simulink model "PSCelecv_2"  (R2020b)
settings: Solver=VariableStepAuto  StartTime=0.0  StopTime=100.0  RelTol=1e-3
undefined symbols (not defined in the file): sigbuilder_block
settings Model: Creator=colpari  LastModifiedBy=colpari

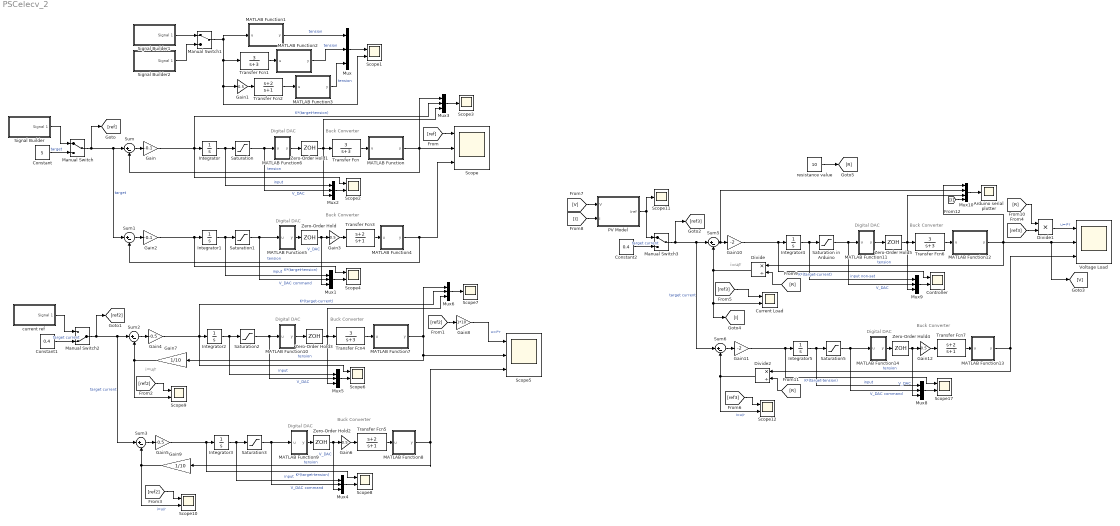
== system PSCelecv_2 ==
  note: i=u/r
  note: Digital DAC
  note: Digital DAC
  note: Buck Converter
  note: Buck Converter
  note: Buck Converter
  note: Digital DAC
  note: Buck Converter
  note: Digital DAC
  note: Buck Converter
  note: Digital DAC
  note: Digital DAC
  note: Buck Converter
  note: i=u/r
  Arduino serial plotter : Scope
  Constant : Constant  Value=5
  Constant1 : Constant  Value=0.4
  Constant2 : Constant  Value=0.4
  Controller : Scope  NumInputPorts=2
  Current Load : Scope  NumInputPorts=2
  Divide : Product  Inputs=*/
  Divide1 : Product  Inputs=**
  Divide2 : Product  Inputs=*/
  Gain : Gain  Gain=-0.1
  Gain{1,3,6,12} (4 alike) : Gain  Gain=0.5
  Gain10 : Gain  Gain=-2
  Gain11 : Gain  Gain=-2
  Gain2 : Gain  Gain=-0.1
  Gain4 : Gain  Gain=-0.5
  Gain5 : Gain  Gain=-0.5
  Gain7 : Gain  Gain=1/10
  Gain8 : Gain  Gain=1*10
  Gain9 : Gain  Gain=1/10
  Integrator{,1..5} (6 alike) : Integrator
  MATLAB Function : MATLAB Function  TreatAsAtomicUnit=on
  MATLAB Function1 : MATLAB Function  TreatAsAtomicUnit=on
  MATLAB Function10 : MATLAB Function  TreatAsAtomicUnit=on
  MATLAB Function11 : MATLAB Function  TreatAsAtomicUnit=on
  MATLAB Function12 : MATLAB Function  TreatAsAtomicUnit=on
  MATLAB Function13 : MATLAB Function  TreatAsAtomicUnit=on
  MATLAB Function14 : MATLAB Function  TreatAsAtomicUnit=on
  MATLAB Function2 : MATLAB Function  TreatAsAtomicUnit=on
  MATLAB Function3 : MATLAB Function  TreatAsAtomicUnit=on
  MATLAB Function4 : MATLAB Function  TreatAsAtomicUnit=on
  MATLAB Function5 : MATLAB Function  TreatAsAtomicUnit=on
  MATLAB Function6 : MATLAB Function  TreatAsAtomicUnit=on
  MATLAB Function7 : MATLAB Function  TreatAsAtomicUnit=on
  MATLAB Function8 : MATLAB Function  TreatAsAtomicUnit=on
  MATLAB Function9 : MATLAB Function  TreatAsAtomicUnit=on
  Manual Switch : ManualSwitch
  Manual Switch1 : ManualSwitch
  Manual Switch2 : ManualSwitch  CurrentSetting=0
  Manual Switch3 : ManualSwitch
  Mux{,1..6,8..9} (9 alike) : Mux  Inputs=3
  Mux10 : Mux
  PV Model : Subsystem
  Saturation{,1..3} (4 alike) : Saturate  UpperLimit=5  LowerLimit=1
  Saturation in Arduino : Saturate  UpperLimit=4.8  LowerLimit=0.2
  Saturation5 : Saturate  UpperLimit=4.8  LowerLimit=0.2
  Scope : Scope  NumInputPorts=3
  Scope{1..2,4,6,8..10,12,17} (9 alike) : Scope  NumInputPorts=2
  Scope11 : Scope
  Scope3 : Scope
  Scope5 : Scope  NumInputPorts=3
  Scope7 : Scope
  Signal Builder : Subsystem  Tag=STV Subsys  LoadFcn=sigbuilder_block('load');  StartFcn=sigbuilder_block('start');  StopFcn=sigbuilder_block('stop');  ClipboardFcn=sigbuilder_block('clipboard');  mask(Sigbuilder block){tuvar=[0:10]}
      mask help: Simulink:masks:SigbuilderBlock_MD
      mask init:
      | if ~strcmp(get_param(bdroot(gcbh),'SimulationStatus'),'stopped') tuvar = sigbuilder_block('maskInit'); end
      settings: CopyFcn=sigbuilder_block('copy');  DeleteFcn=sigbuilder_block('delete');  ModelCloseFcn=sigbuilder_block('modelClose');  PreSaveFcn=sigbuilder_block('preSave');  PauseFcn=sigbuilder_block('pause');  ContinueFcn=sigbuilder_block('continue');  NameChangeFcn=sigbuilder_block('namechange');  OpenFcn=sigbuilder_block('open',[337.5 87.75 550.5 399.75 ]);  CloseFcn=sigbuilder_block('close');
      mask Display: plot(0, 0, 100, 100,[2, 2, 32, 32, 2], [68, 8, 8, 68, 68],[32, 2], [38, 38], [32, 19, 2],[53, 60, 44], [32, 17, 17, 2],[16, 16, 31, 31]);txt = getActiveGroup(gcbh);text(2, 100, txt,'verticalAlignment', 'top');
  Signal Builder1 : Subsystem  Tag=STV Subsys  LoadFcn=sigbuilder_block('load');  StartFcn=sigbuilder_block('start');  StopFcn=sigbuilder_block('stop');  ClipboardFcn=sigbuilder_block('clipboard');  mask(Sigbuilder block){tuvar=[0:10]}
      mask help: Simulink:masks:SigbuilderBlock_MD
      mask init:
      | if ~strcmp(get_param(bdroot(gcbh),'SimulationStatus'),'stopped') tuvar = sigbuilder_block('maskInit'); end
      settings: CopyFcn=sigbuilder_block('copy');  DeleteFcn=sigbuilder_block('delete');  ModelCloseFcn=sigbuilder_block('modelClose');  PreSaveFcn=sigbuilder_block('preSave');  PauseFcn=sigbuilder_block('pause');  ContinueFcn=sigbuilder_block('continue');  NameChangeFcn=sigbuilder_block('namechange');  OpenFcn=sigbuilder_block('open',[437.6 199.2 550.4 400 ]);  CloseFcn=sigbuilder_block('close');
      mask Display: plot(0, 0, 100, 100,[2, 2, 32, 32, 2], [68, 8, 8, 68, 68],[32, 2], [38, 38], [32, 19, 2],[53, 60, 44], [32, 17, 17, 2],[16, 16, 31, 31]);txt = getActiveGroup(gcbh);text(2, 100, txt,'verticalAlignment', 'top');
  Signal Builder2 : Subsystem  Tag=STV Subsys  LoadFcn=sigbuilder_block('load');  StartFcn=sigbuilder_block('start');  StopFcn=sigbuilder_block('stop');  ClipboardFcn=sigbuilder_block('clipboard');  mask(Sigbuilder block){tuvar=[0:10]}
      mask help: Simulink:masks:SigbuilderBlock_MD
      mask init:
      | if ~strcmp(get_param(bdroot(gcbh),'SimulationStatus'),'stopped') tuvar = sigbuilder_block('maskInit'); end
      settings: CopyFcn=sigbuilder_block('copy');  DeleteFcn=sigbuilder_block('delete');  ModelCloseFcn=sigbuilder_block('modelClose');  PreSaveFcn=sigbuilder_block('preSave');  PauseFcn=sigbuilder_block('pause');  ContinueFcn=sigbuilder_block('continue');  NameChangeFcn=sigbuilder_block('namechange');  OpenFcn=sigbuilder_block('open',[337.5 87.75 550.5 399.75 ]);  CloseFcn=sigbuilder_block('close');
      mask Display: plot(0, 0, 100, 100,[2, 2, 32, 32, 2], [68, 8, 8, 68, 68],[32, 2], [38, 38], [32, 19, 2],[53, 60, 44], [32, 17, 17, 2],[16, 16, 31, 31]);txt = getActiveGroup(gcbh);text(2, 100, txt,'verticalAlignment', 'top');
  Sum{,1..3,5..6} (6 alike) : Sum  Inputs=|+-
  Transfer Fcn{,1,4,6} (4 alike) : TransferFcn  Numerator=[3]  Denominator=[1 3]
  Transfer Fcn{2..3,5,7} (4 alike) : TransferFcn  Numerator=[1 2]  Denominator=[1 1]
  Voltage Load : Scope  NumInputPorts=3
  Zero-Order Hold{,1..5} (6 alike) : ZeroOrderHold  SampleTime=0.05
  current ref : Subsystem  Tag=STV Subsys  LoadFcn=sigbuilder_block('load');  StartFcn=sigbuilder_block('start');  StopFcn=sigbuilder_block('stop');  ClipboardFcn=sigbuilder_block('clipboard');  mask(Sigbuilder block){tuvar=[0:10]}
      mask help: Simulink:masks:SigbuilderBlock_MD
      mask init:
      | if ~strcmp(get_param(bdroot(gcbh),'SimulationStatus'),'stopped') tuvar = sigbuilder_block('maskInit'); end
      settings: CopyFcn=sigbuilder_block('copy');  DeleteFcn=sigbuilder_block('delete');  ModelCloseFcn=sigbuilder_block('modelClose');  PreSaveFcn=sigbuilder_block('preSave');  PauseFcn=sigbuilder_block('pause');  ContinueFcn=sigbuilder_block('continue');  NameChangeFcn=sigbuilder_block('namechange');  OpenFcn=sigbuilder_block('open',[5.4 30 1141.2 594.6 ]);  CloseFcn=sigbuilder_block('close');
      mask Display: plot(0, 0, 100, 100,[2, 2, 32, 32, 2], [68, 8, 8, 68, 68],[32, 2], [38, 38], [32, 19, 2],[53, 60, 44], [32, 17, 17, 2],[16, 16, 31, 31]);txt = getActiveGroup(gcbh);text(2, 100, txt,'verticalAlignment', 'top');
  resistance value : Constant  Value=10
  wires:
  MATLAB Function/1(y) -> Mux3/1, Scope/2, Sum/2  "tension"
  Sum/1 -> Gain/1
  Transfer Fcn/1 -> MATLAB Function/1(u)
  Signal Builder/1(Signal 1) -> Manual Switch/1
  MATLAB Function1/1(y) -> Mux/1  "tension"
  Manual Switch1/1 -> Scope1/2, Gain1/1, Transfer Fcn1/1, MATLAB Function1/1(u)
  Transfer Fcn1/1 -> MATLAB Function2/1(u)
  MATLAB Function2/1(y) -> Mux/2  "tension"
  Constant/1 -> Manual Switch/2  "target"
  Gain/1 -> Mux3/2, Scope2/1, Integrator/1  "K*(target-tension)"
  Saturation/1 -> Mux2/2, MATLAB Function6/1(u)  "V_DAC"
  Mux/1 -> Scope1/1
  Integrator/1 -> Mux2/1, Saturation/1  "input"
  Signal Builder1/1(Signal 1) -> Manual Switch1/1
  Signal Builder2/1(Signal 1) -> Manual Switch1/2
  Transfer Fcn2/1 -> MATLAB Function3/1(u)
  MATLAB Function3/1(y) -> Mux/3  "tension"
  Gain1/1 -> Transfer Fcn2/1
  MATLAB Function4/1(y) -> Scope/3, Sum1/2  "tension"
  Saturation1/1 -> MATLAB Function5/1(u), Mux1/2  "V_DAC command"
  Sum1/1 -> Gain2/1
  Gain2/1 -> Scope4/1, Integrator1/1  "K*(target-tension)"
  Integrator1/1 -> Mux1/1, Saturation1/1  "input"
  Transfer Fcn3/1 -> MATLAB Function4/1(u)
  Manual Switch/1 -> [ref], Sum1/1, Sum/1  "target"
  Gain3/1 -> Transfer Fcn3/1
  [ref] -> Scope/1
  MATLAB Function5/1(y) -> Zero-Order Hold/1
  Zero-Order Hold/1 -> Mux1/3, Gain3/1  "V_DAC"
  MATLAB Function6/1(y) -> Zero-Order Hold1/1
  Zero-Order Hold1/1 -> Mux3/3, Mux2/3, Transfer Fcn/1
  Mux1/1 -> Scope4/2
  Mux2/1 -> Scope2/2
  Mux3/1 -> Scope3/1
  Transfer Fcn5/1 -> MATLAB Function8/1(u)
  Transfer Fcn4/1 -> MATLAB Function7/1(u)
  Mux5/1 -> Scope6/2
  Gain5/1 -> Scope8/1, Integrator3/1  "K*(target-tension)"
  MATLAB Function9/1(y) -> Zero-Order Hold2/1
  [ref2] -> Gain8/1
  Gain6/1 -> Transfer Fcn5/1
  Zero-Order Hold2/1 -> Mux4/3, Gain6/1  "V_DAC"
  Manual Switch2/1 -> [ref2], Sum3/1, Sum2/1  "target current"
  Gain4/1 -> Mux6/2, Scope6/1, Integrator2/1  "K*(target-current)"
  Saturation3/1 -> MATLAB Function9/1(u), Mux4/2  "V_DAC command"
  MATLAB Function8/1(y) -> Scope5/3, Gain9/1  "tension"
  Sum3/1 -> Gain5/1
  Constant1/1 -> Manual Switch2/2  "target current"
  Integrator2/1 -> Mux5/1, Saturation2/1  "input"
  Saturation2/1 -> Mux5/2, MATLAB Function10/1(u)  "V_DAC"
  Integrator3/1 -> Mux4/1, Saturation3/1  "input"
  MATLAB Function10/1(y) -> Zero-Order Hold3/1
  Mux4/1 -> Scope8/2
  current ref/1(Signal 1) -> Manual Switch2/1
  Sum2/1 -> Gain4/1
  MATLAB Function7/1(y) -> Gain7/1, Scope5/2, Mux6/1  "tension"
  Zero-Order Hold3/1 -> Mux6/3, Mux5/3, Transfer Fcn4/1
  Gain7/1 -> Scope9/2, Sum2/2
  Mux6/1 -> Scope7/1
  [ref2] -> Scope9/1
  Gain8/1 -> Scope5/1  "u=i*r"
  Gain9/1 -> Scope10/2, Sum3/2  "i=u/r"
  [ref2] -> Scope10/1
  [I] -> PV Model/2(I)
  [V] -> PV Model/1(V)
  [ref3] -> Current Load/1
  [ref3] -> Divide1/2
  Zero-Order Hold5/1 -> Mux10/3, Mux9/3, Transfer Fcn6/1
  PV Model/1(Iref) -> Manual Switch3/1, Scope11/1
  MATLAB Function11/1(y) -> Zero-Order Hold5/1
  MATLAB Function12/1(y) -> Divide/1, Mux10/1, [V], Voltage Load/2  "tension"
  Saturation in Arduino/1 -> Mux9/2, MATLAB Function11/1(u)  "V_DAC"
  Divide/1 -> Sum5/2, [I], Current Load/2
  Mux8/1 -> Scope17/2
  Integrator5/1 -> Mux8/1, Saturation5/1  "input"
  Integrator4/1 -> Mux9/1, Saturation in Arduino/1  "input non-sat"
  Constant2/1 -> Manual Switch3/2  "target current"
  MATLAB Function13/1(y) -> Divide2/1, Voltage Load/3  "tension"
  Divide1/1 -> Voltage Load/1  "u=i*r"
  Sum6/1 -> Gain11/1
  [ref3] -> Scope12/1
  Saturation5/1 -> MATLAB Function14/1(u), Mux8/2  "V_DAC command"
  Zero-Order Hold4/1 -> Mux8/3, Gain12/1  "V_DAC"
  Sum5/1 -> Mux10/2, Gain10/1
  Divide2/1 -> Sum6/2, Scope12/2  "i=u/r"
  Gain12/1 -> Transfer Fcn7/1
  Mux10/1 -> Arduino serial plotter/1
  Transfer Fcn7/1 -> MATLAB Function13/1(u)
  Mux9/1 -> Controller/2
  MATLAB Function14/1(y) -> Zero-Order Hold4/1
  Manual Switch3/1 -> [ref3], Sum6/1, Sum5/1  "target current"
  Transfer Fcn6/1 -> MATLAB Function12/1(u)
  Gain11/1 -> Scope17/1, Integrator5/1  "K*(target-tension)"
  Gain10/1 -> Controller/1, Integrator4/1  "K*(target-current)"
  resistance value/1 -> [R]
  [R] -> Divide/2
  [R] -> Divide1/1
  [R] -> Divide2/2
  [I] -> Mux10/4

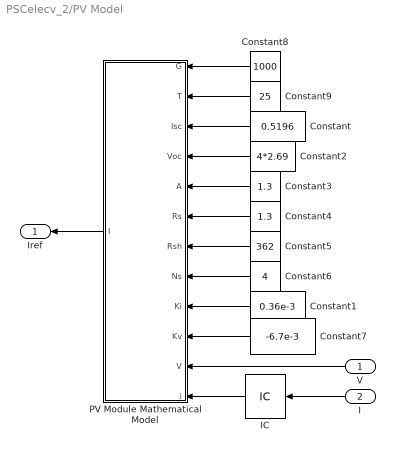
== system PSCelecv_2/PV Model ==
  V : Inport
  I : Inport  Port=2
  Constant : Constant  Value=0.5196
  Constant1 : Constant  Value=0.36e-3
  Constant2 : Constant  Value=4*2.69
  Constant3 : Constant  Value=1.3
  Constant4 : Constant  Value=1.3
  Constant5 : Constant  Value=362
  Constant6 : Constant  Value=4
  Constant7 : Constant  Value=-6.7e-3
  Constant8 : Constant  Value=1000
  Constant9 : Constant  Value=25
  IC : InitialCondition  Value=0
  PV Module Mathematical Model : MATLAB Function  TreatAsAtomicUnit=on
  Iref : Outport
  wires:
  Constant/1 -> PV Module Mathematical Model/3(Isc)
  Constant7/1 -> PV Module Mathematical Model/10(Kv)
  Constant5/1 -> PV Module Mathematical Model/7(Rsh)
  Constant6/1 -> PV Module Mathematical Model/8(Ns)
  Constant1/1 -> PV Module Mathematical Model/9(Ki)
  Constant8/1 -> PV Module Mathematical Model/1(G)
  Constant4/1 -> PV Module Mathematical Model/6(Rs)
  Constant2/1 -> PV Module Mathematical Model/4(Voc)
  Constant9/1 -> PV Module Mathematical Model/2(T)
  Constant3/1 -> PV Module Mathematical Model/5(A)
  PV Module Mathematical Model/1(I) -> Iref/1
  I/1 -> IC/1
  IC/1 -> PV Module Mathematical Model/12(i)
  V/1 -> PV Module Mathematical Model/11(V)

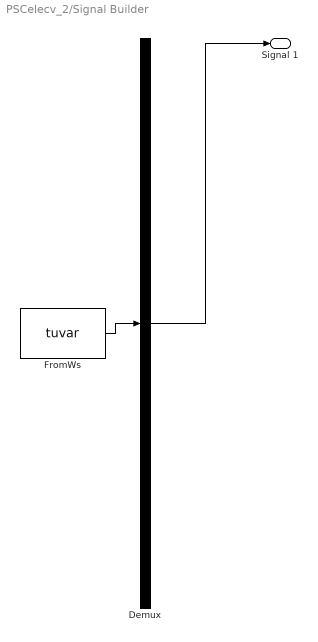
== system PSCelecv_2/Signal Builder ==
  Demux : Demux  Tag=STV Demux  Outputs=1
      settings: DisplayOption=none
  FromWs : FromWorkspace  Tag=STV FromWs  VariableName=tuvar
      SigBuilderData=|
      | common.afterFinalStr = 'Extrapolate'
      | common.sampleTime = 0
      | dataSet.timeRange = [0 10]
      | dataSet.name = 'Group 1'
      | sbobj.Groups.Name = 'Group 1'
      | sbobj.Groups.Signals.Name = 'Signal 1'
      | sbobj.Groups.Signals.XData = [0 4 4 6 6 10]
      | sbobj.Groups.Signals.YData = [0 5 -0.02 1 0 0]
  Signal 1 : Outport  Tag=STV Outport
  wires:
  Demux/1 -> Signal 1/1
  FromWs/1 -> Demux/1

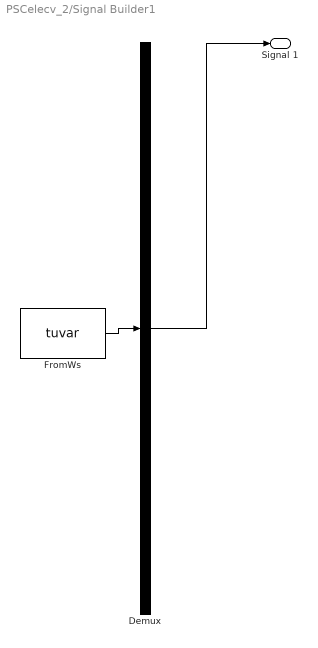
== system PSCelecv_2/Signal Builder1 ==
  Demux : Demux  Tag=STV Demux  Outputs=1
      settings: DisplayOption=none
  FromWs : FromWorkspace  Tag=STV FromWs  VariableName=tuvar
      SigBuilderData=|
      | common.afterFinalStr = 'Extrapolate'
      | common.sampleTime = 0
      | dataSet.timeRange = [0 100]
      | dataSet.name = 'Group 1'
      | sbobj.Groups.Name = 'Group 1'
      | sbobj.Groups.Signals.Name = 'Signal 1'
      | sbobj.Groups.Signals.XData = [0 30 30 40 50 60 90 100]
      | sbobj.Groups.Signals.YData = [0 5 0 1 0 3 0 0]
      | sbobj.Groups.TimeRange = [0 100]
  Signal 1 : Outport  Tag=STV Outport
  wires:
  Demux/1 -> Signal 1/1
  FromWs/1 -> Demux/1

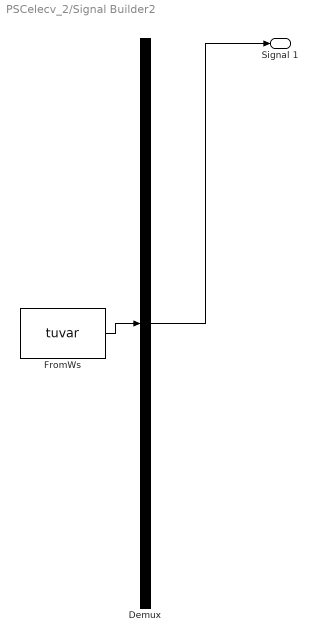
== system PSCelecv_2/Signal Builder2 ==
  Demux : Demux  Tag=STV Demux  Outputs=1
      settings: DisplayOption=none
  FromWs : FromWorkspace  Tag=STV FromWs  VariableName=tuvar
      SigBuilderData=|
      | common.afterFinalStr = 'Extrapolate'
      | common.sampleTime = 0
      | dataSet.timeRange = [0 10]
      | dataSet.name = 'Group 1'
      | sbobj.Groups.Name = 'Group 1'
      | sbobj.Groups.Signals.Name = 'Signal 1'
      | sbobj.Groups.Signals.XData = [0 4 4 6 6 10]
      | sbobj.Groups.Signals.YData = [0 5 -0.02 1 0 0]
  Signal 1 : Outport  Tag=STV Outport
  wires:
  Demux/1 -> Signal 1/1
  FromWs/1 -> Demux/1

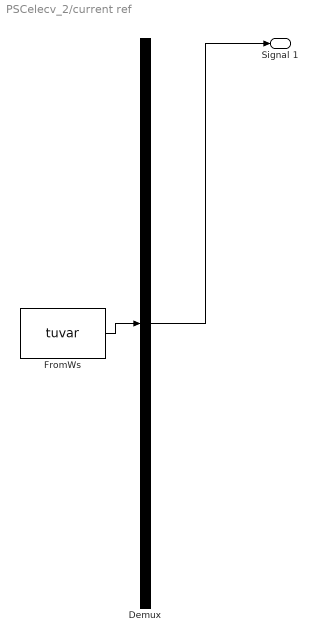
== system PSCelecv_2/current ref ==
  Demux : Demux  Tag=STV Demux  Outputs=1
      settings: DisplayOption=none
  FromWs : FromWorkspace  Tag=STV FromWs  VariableName=tuvar
      SigBuilderData=|
      | common.afterFinalStr = 'Extrapolate'
      | common.sampleTime = 0
      | dataSet.timeRange = [0 10]
      | dataSet.name = 'Group 1'
      | sbobj.Groups.Name = 'Group 1'
      | sbobj.Groups.Signals.Name = 'Signal 1'
      | sbobj.Groups.Signals.XData = [0 4 4 6 7 9 10]
      | sbobj.Groups.Signals.YData = [0 0.5 0.1 1 0.2 0.1 0.1]
  Signal 1 : Outport  Tag=STV Outport
  wires:
  Demux/1 -> Signal 1/1
  FromWs/1 -> Demux/1

== matlab function PSCelecv_2/MATLAB Function11 ==
  data: u input; y output
function y = fcn(u)
edges=0:1/4095:5;
y = discretize(u,edges)/4096;

== matlab function PSCelecv_2/MATLAB Function12 ==
  data: u input; y output
function y = fcn(u)

y = 16-2.9414*u;

== matlab function PSCelecv_2/MATLAB Function13 ==
  data: u input; y output
function y = fcn(u)

y = 16-2.9414*u;

== matlab function PSCelecv_2/MATLAB Function14 ==
  data: u input; y output
function y = fcn(u)
edges=0:1/4095:5;
y = discretize(u,edges)/4096;

== matlab function PSCelecv_2/MATLAB Function1 ==
  data: u input; y output
function y = fcn(u)

y = 16-2.9414*u;

== matlab function PSCelecv_2/MATLAB Function ==
  data: u input; y output
function y = fcn(u)

y = 16-2.9414*u;

== matlab function PSCelecv_2/MATLAB Function2 ==
  data: u input; y output
function y = fcn(u)

y = 16-2.9414*u;

== matlab function PSCelecv_2/MATLAB Function3 ==
  data: u input; y output
function y = fcn(u)

y = 16-2.9414*u;

== matlab function PSCelecv_2/MATLAB Function4 ==
  data: u input; y output
function y = fcn(u)

y = 16-2.9414*u;

== matlab function PSCelecv_2/MATLAB Function5 ==
  data: u input; y output
function y = fcn(u)
edges=0:1/4095:5;
y = discretize(u,edges)/4096;

== matlab function PSCelecv_2/MATLAB Function6 ==
  data: u input; y output
function y = fcn(u)
edges=0:1/4095:5;
y = discretize(u,edges)/4096;

== matlab function PSCelecv_2/MATLAB Function10 ==
  data: u input; y output
function y = fcn(u)
edges=0:1/4095:5;
y = discretize(u,edges)/4096;

== matlab function PSCelecv_2/MATLAB Function7 ==
  data: u input; y output
function y = fcn(u)

y = 16-2.9414*u;

== matlab function PSCelecv_2/MATLAB Function8 ==
  data: u input; y output
function y = fcn(u)

y = 16-2.9414*u;

== matlab function PSCelecv_2/MATLAB Function9 ==
  data: u input; y output
function y = fcn(u)
edges=0:1/4095:5;
y = discretize(u,edges)/4096;

== matlab function PSCelecv_2/PV Model/PV Module Mathematical Model ==
  data: G input; T input; Isc input; Voc input; A input; Rs input; Rsh input; Ns input; Ki input; Kv input; V input; i input; I output
function I = fcn(G,T,Isc,Voc,A,Rs,Rsh,Ns,Ki,Kv,V,i)
    
    q = 1.6e-19;                          % Electron charge
    k = 1.38e-23;                         % Boltzmann constant
    Tcell = 273+T;                        % Cell temperature in Kelvin
    vt=(A*k*Tcell*Ns)/q;                  % Thermal voltage Equation(5)
        
    Isc_T = Isc+((Isc*(Ki/100))*(T-25));  % Isc temperature coef Equation(6)
    Voc_T = Voc+((Voc*(Kv/100))*(T-25));  % Voc temperature coef Equation(7)
    Is = Isc_T/(exp(Voc_T/vt)-1);         % Reverse saturation current Equation(8)
    Iph = Isc_T*(G/1000);                 % Photon current Equation(9)
    
    % Single diode model output current Equation(4)
    I = Iph-(Is*(exp((V+(i*Rs))/vt)-1))-((V+(i*Rs))/Rsh);
    I(I < 0) = 0;
end
